simulink model "simu_25a"  (R2025a)
settings: Solver=ode4  StartTime=0.0  StopTime=15  FixedStep=0.01  RelTol=1e-3
libraries: simulink_extras x4, simulink x1
settings Model: Creator=psp_dada  LastModifiedBy=psp_dada

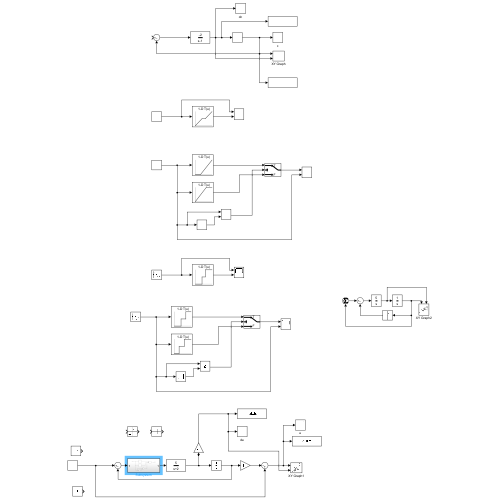
[thumbnail: Simulink's stored preview of the top-level diagram]
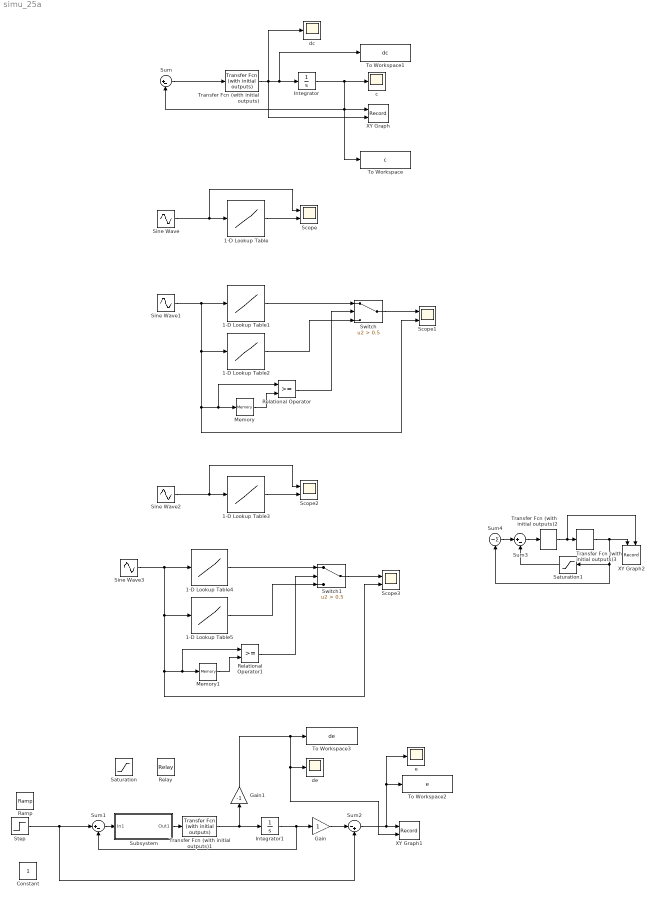
== system simu_25a ==
  1-D Lookup Table : Lookup_n-D  NumberOfTableDimensions=1  BreakpointsForDimension1=[-5 -1 1 5]  Table=[-4 0 0 4]  InternalRulePriority=Speed  RndMeth=Simplest
  1-D Lookup Table1 : Lookup_n-D  NumberOfTableDimensions=1  BreakpointsForDimension1=[-3 -1 3]  Table=[-1 -1 1]  InternalRulePriority=Speed  RndMeth=Simplest
  1-D Lookup Table2 : Lookup_n-D  NumberOfTableDimensions=1  BreakpointsForDimension1=[-3 1 3]  Table=[-1 1 1]  InternalRulePriority=Speed  RndMeth=Simplest
  1-D Lookup Table3 : Lookup_n-D  NumberOfTableDimensions=1  BreakpointsForDimension1=[-5 -1.001 -1 1 1.001 5]  Table=[-1 -1 0 0 1 1]  InternalRulePriority=Speed  RndMeth=Simplest
  1-D Lookup Table4 : Lookup_n-D  NumberOfTableDimensions=1  BreakpointsForDimension1=[-5 -1.001 -1 2 2.001 5]  Table=[-1 -1 0 0 1 1]  InternalRulePriority=Speed  RndMeth=Simplest
  1-D Lookup Table5 : Lookup_n-D  NumberOfTableDimensions=1  BreakpointsForDimension1=[-5 -2.0001 -2 1 1.001 5]  Table=[-1 -1 0 0 1 1]  InternalRulePriority=Speed  RndMeth=Simplest
  Constant : Constant
  Gain : Gain
  Gain1 : Gain  Gain=-1
  Integrator : Integrator  InitialCondition=10
  Integrator1 : Integrator  InitialCondition=-0.5
  Memory : Memory
  Memory1 : Memory
  Ramp : simulink/Sources/Ramp  slope=1  start=0  InitialOutput=0
  Relational Operator : RelationalOperator  OutDataTypeStr=boolean  RndMeth=Simplest  InputSameDT=off
  Relational Operator1 : RelationalOperator  OutDataTypeStr=boolean  RndMeth=Simplest  InputSameDT=off
  Relay : Relay  OnSwitchValue=1  OffSwitchValue=-1  OffOutputValue=-1
  Saturation : Saturate
  Saturation1 : Saturate  UpperLimit=1  LowerLimit=-1
  Scope{,1..3} (4 alike) : Scope  NumInputPorts=2
      Scope settings: ActiveDisplayYMinimum=-2.4929308281295746  ActiveDisplayYMaximum=2.498743705676405  DataLoggingVariableName=ScopeData2
      Scope1 settings: ActiveDisplayYMinimum=-3.747506879253339  ActiveDisplayYMaximum=3.7490167404100494  DataLoggingVariableName=ScopeData3
      Scope2 settings: ActiveDisplayYMinimum=-2.4929308281295746  ActiveDisplayYMaximum=2.498743705676405  DataLoggingVariableName=ScopeData4
      Scope3 settings: ActiveDisplayYMinimum=-2.4983379195022257  ActiveDisplayYMaximum=2.4993444936066997  DataLoggingVariableName=ScopeData5
  Sine Wave : Sin  Amplitude=2  SampleTime=0
  Sine Wave1 : Sin  Amplitude=3  SampleTime=0
  Sine Wave2 : Sin  Amplitude=2  SampleTime=0
  Sine Wave3 : Sin  Amplitude=2  SampleTime=0
  Step : Step  Time=0  After=0  SampleTime=0
  Subsystem : Subsystem
  Sum : Sum  Inputs=|+-
  Sum1 : Sum  Inputs=|+-
  Sum2 : Sum  Inputs=|-+
  Sum3 : Sum  Inputs=|+-
  Sum4 : Sum  Inputs=||-
  Switch : Switch  Criteria=u2 > Threshold  Threshold=0.5  SaturateOnIntegerOverflow=off  InputSameDT=off
  Switch1 : Switch  Criteria=u2 > Threshold  Threshold=0.5  SaturateOnIntegerOverflow=off  InputSameDT=off
  To Workspace : ToWorkspace  VariableName=c  SampleTime=-1
  To Workspace1 : ToWorkspace  VariableName=dc  SampleTime=-1
  To Workspace2 : ToWorkspace  VariableName=e  SampleTime=-1
  To Workspace3 : ToWorkspace  VariableName=de  SampleTime=-1
  Transfer Fcn (with initial outputs) : simulink_extras/Additional Linear/Transfer Fcn (with initial outputs)  N=[-2]  D=[1 -1]  Y0=-10.5  U0=0
  Transfer Fcn (with initial outputs)1 : simulink_extras/Additional Linear/Transfer Fcn (with initial outputs)  N=[5]  D=[1 2]  Y0=0.3  U0=0
  Transfer Fcn (with initial outputs)2 : simulink_extras/Additional Linear/Transfer Fcn (with initial outputs)  N=[5]  D=[1 0]  Y0=2  U0=0
  Transfer Fcn (with initial outputs)3 : simulink_extras/Additional Linear/Transfer Fcn (with initial outputs)  N=[1]  D=[1 0]  Y0=2  U0=0
  XY Graph : Record  NumPorts=2.0  FileSettingsInternal="{\"entries\":[{\"content\":{\"excelSettings\":{\"content\":{},\"type\":\"Streamout.ExcelSettings\"},\"parquetSettings\":{\"content\":{},\"type\":\"Streamout.ParquetSettings\"}},\"type\":\"Streamout.FileSettingStorage\",\"uuid\":\"\"}],\"packageUris\":[\"http:\\/\\/schema.mathworks.com\\/mf0\\/streamout_blocks\\/R2020a\"],\"version\":\"1.0\"}"  FrameSettings=[0, 0]  Layout=[1 1]  SignalsInternal="{\"entries\":[{\"content\":{\"signals\":[{\"content\":{\"blockPath\":[],\"dimensions\":[1],\"domain\":\"\",\"lineColor\":\"#a2142f\",\"plots\":[ 1 ],\"port\":1,\"signalID\":1,\"signalName\":\"Integrator\"},\"type\":\"RecordBlkView.Signal\",\"uuid\":\"\"},{\"content\":{\"blockPath\":[],\"dimensions\":[1],\"domain\":\"\",\"lineColor\":\"#139fff\",\"plots\":[ 1 ],\"port\":2,\"signalID\":2,\"signalName\":\"Transfer Fcn\\n(with initial outputs)\"},\"type\":\"RecordBlkView.Signal\",\"uuid\":\"\"}]},\"type\":\"RecordBlkView.InputSignals\",\"uuid\":\"\"}],\"packageUris\":[\"http:\\/\\/schema.mathworks.com\\/mf0\\/streamout_blocks\\/R2020a\"],\"version\":\"1.0\"}"  VisualizationBindings="{\"xyplotplugin\":{\"info\":[{\"series\":[{\"bindingParametersList\":[{\"parameter\":\"X-Axis\",\"signalID\":1,\"signalName\":\"Integrator\"},{\"parameter\":\"Y-Axis\",\"signalID\":2,\"signalName\":\"Transfer Fcn\\n(with initial outputs)\"}],\"seriesID\":0}],\"subplotID\":1}]}}"  CompatibilityTag=XY
  XY Graph1 : Record  NumPorts=2.0  FileSettingsInternal="{\"entries\":[{\"content\":{\"excelSettings\":{\"content\":{},\"type\":\"Streamout.ExcelSettings\"},\"parquetSettings\":{\"content\":{},\"type\":\"Streamout.ParquetSettings\"}},\"type\":\"Streamout.FileSettingStorage\",\"uuid\":\"\"}],\"packageUris\":[\"http:\\/\\/schema.mathworks.com\\/mf0\\/streamout_blocks\\/R2020a\"],\"version\":\"1.0\"}"  FrameSettings=[0, 0]  Layout=[1 1]  SignalsInternal="{\"entries\":[{\"content\":{\"signals\":[{\"content\":{\"blockPath\":[],\"dimensions\":[1],\"domain\":\"\",\"lineColor\":\"#a2142f\",\"plots\":[ 1 ],\"port\":1,\"signalID\":1,\"signalName\":\"Sum2\"},\"type\":\"RecordBlkView.Signal\",\"uuid\":\"\"},{\"content\":{\"blockPath\":[],\"dimensions\":[1],\"domain\":\"\",\"lineColor\":\"#139fff\",\"plots\":[ 1 ],\"port\":2,\"signalID\":2,\"signalName\":\"Gain1\"},\"type\":\"RecordBlkView.Signal\",\"uuid\":\"\"}]},\"type\":\"RecordBlkView.InputSignals\",\"uuid\":\"\"}],\"packageUris\":[\"http:\\/\\/schema.mathworks.com\\/mf0\\/streamout_blocks\\/R2020a\"],\"version\":\"1.0\"}"  VisualizationBindings="{\"xyplotplugin\":{\"info\":[{\"series\":[{\"bindingParametersList\":[{\"parameter\":\"X-Axis\",\"signalID\":1,\"signalName\":\"Sum2\"},{\"parameter\":\"Y-Axis\",\"signalID\":2,\"signalName\":\"Gain1\"}],\"seriesID\":0}],\"subplotID\":1}]}}"  CompatibilityTag=XY
  XY Graph2 : Record  NumPorts=2.0  FileSettingsInternal="{\"entries\":[{\"content\":{\"excelSettings\":{\"content\":{},\"type\":\"Streamout.ExcelSettings\"},\"parquetSettings\":{\"content\":{},\"type\":\"Streamout.ParquetSettings\"}},\"type\":\"Streamout.FileSettingStorage\",\"uuid\":\"\"}],\"packageUris\":[\"http:\\/\\/schema.mathworks.com\\/mf0\\/streamout_blocks\\/R2020a\"],\"version\":\"1.0\"}"  FrameSettings=[0, 0]  Layout=[1 1]  SignalsInternal="{\"entries\":[{\"content\":{\"signals\":[{\"content\":{\"blockPath\":[],\"dimensions\":[1],\"domain\":\"\",\"lineColor\":\"#a2142f\",\"plots\":[ 1 ],\"port\":1,\"signalID\":1,\"signalName\":\"Transfer Fcn\\n(with initial outputs)3\"},\"type\":\"RecordBlkView.Signal\",\"uuid\":\"\"},{\"content\":{\"blockPath\":[],\"dimensions\":[1],\"domain\":\"\",\"lineColor\":\"#139fff\",\"plots\":[ 1 ],\"port\":2,\"signalID\":2,\"signalName\":\"Transfer Fcn\\n(with initial outputs)2\"},\"type\":\"RecordBlkView.Signal\",\"uuid\":\"\"}]},\"type\":\"RecordBlkView.InputSignals\",\"uuid\":\"\"}],\"packageUris\":[\"http:\\/\\/schema.mathworks.com\\/mf0\\/streamout_blocks\\/R2020a\"],\"version\":\"1.0\"}"  VisualizationBindings="{\"xyplotplugin\":{\"info\":[{\"series\":[{\"bindingParametersList\":[{\"parameter\":\"X-Axis\",\"signalID\":1,\"signalName\":\"Transfer Fcn\\n(with initial outputs)3\"},{\"parameter\":\"Y-Axis\",\"signalID\":2,\"signalName\":\"Transfer Fcn\\n(with initial outputs)2\"}],\"seriesID\":0}],\"subplotID\":1}]}}"  CompatibilityTag=XY
  c : Scope
      settings: ActiveDisplayYMinimum=-1  ActiveDisplayYMaximum=1
  dc : Scope
      settings: ActiveDisplayYMinimum=-1  ActiveDisplayYMaximum=1
  de : Scope
      settings: ActiveDisplayYMinimum=-2.9388413485397145  ActiveDisplayYMaximum=2.9377251379229867  DataLoggingVariableName=ScopeData7
  e : Scope
      settings: ActiveDisplayYMinimum=-1.6884338081502135  ActiveDisplayYMaximum=1.6894637241988331  DataLoggingVariableName=ScopeData6
  wires:
  Sum/1 -> Transfer Fcn (with initial outputs)/1
  Transfer Fcn (with initial outputs)/1 -> dc/1, XY Graph/2, To Workspace1/1, Integrator/1
  Integrator/1 -> Sum/2, To Workspace/1, XY Graph/1, c/1
  Sine Wave/1 -> 1-D Lookup Table/1, Scope/1
  1-D Lookup Table/1 -> Scope/2
  Sine Wave1/1 -> 1-D Lookup Table2/1, Relational Operator/1, Memory/1, Scope1/2, 1-D Lookup Table1/1
  1-D Lookup Table1/1 -> Switch/1
  Switch/1 -> Scope1/1
  1-D Lookup Table2/1 -> Switch/3
  Relational Operator/1 -> Switch/2
  Memory/1 -> Relational Operator/2
  Sine Wave2/1 -> 1-D Lookup Table3/1, Scope2/1
  1-D Lookup Table3/1 -> Scope2/2
  Sine Wave3/1 -> 1-D Lookup Table5/1, Relational Operator1/1, Memory1/1, Scope3/2, 1-D Lookup Table4/1
  1-D Lookup Table5/1 -> Switch1/3
  1-D Lookup Table4/1 -> Switch1/1
  Relational Operator1/1 -> Switch1/2
  Switch1/1 -> Scope3/1
  Memory1/1 -> Relational Operator1/2
  Step/1 -> Sum2/2, Sum1/1
  Sum1/1 -> Subsystem/1(In1)
  Subsystem/1(Out1) -> Transfer Fcn (with initial outputs)1/1
  Transfer Fcn (with initial outputs)1/1 -> Integrator1/1, Gain1/1
  Integrator1/1 -> Sum1/2, Gain/1
  Gain1/1 -> XY Graph1/2, de/1, To Workspace3/1
  Gain/1 -> Sum2/1
  Sum2/1 -> To Workspace2/1, e/1, XY Graph1/1
  Saturation1/1 -> Sum3/2
  Sum4/1 -> Sum3/1
  Transfer Fcn (with initial outputs)3/1 -> XY Graph2/1, Sum4/1, Saturation1/1
  Transfer Fcn (with initial outputs)2/1 -> Transfer Fcn (with initial outputs)3/1, XY Graph2/2
  Sum3/1 -> Transfer Fcn (with initial outputs)2/1

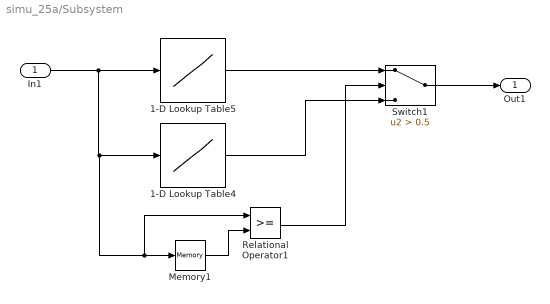
== system simu_25a/Subsystem ==
  In1 : Inport
  1-D Lookup Table4 : Lookup_n-D  NumberOfTableDimensions=1  BreakpointsForDimension1=[-2 -1.001 -1 2]  Table="[-1 -1  1 1]"  InternalRulePriority=Speed  RndMeth=Simplest
  1-D Lookup Table5 : Lookup_n-D  NumberOfTableDimensions=1  BreakpointsForDimension1=[-2 1 1.001 2]  Table=[-1 -1 1 1]  InternalRulePriority=Speed  RndMeth=Simplest
  Memory1 : Memory
  Relational Operator1 : RelationalOperator  OutDataTypeStr=boolean  RndMeth=Simplest  InputSameDT=off
  Switch1 : Switch  Criteria=u2 > Threshold  Threshold=0.5  SaturateOnIntegerOverflow=off  InputSameDT=off
  Out1 : Outport
  wires:
  In1/1 -> 1-D Lookup Table5/1, 1-D Lookup Table4/1, Relational Operator1/1, Memory1/1
  Memory1/1 -> Relational Operator1/2
  1-D Lookup Table5/1 -> Switch1/1
  Relational Operator1/1 -> Switch1/2
  Switch1/1 -> Out1/1
  1-D Lookup Table4/1 -> Switch1/3
